simulink model "dynamic_simulation_synth_admittance_alone_2020a"  (R2020a)
settings: Solver=FixedStepAuto  StartTime=time_start  StopTime=time_end  FixedStep=dt  RelTol=1e-3
values from neighbouring files (symbols this model uses):
  B = 10    [hinfCostFunc.m]    (also in hinf_analysis_z.m; hinf_cmd_lmi.m = [zeros(4,2); Sigma.B]; init_rob_synth_sim.m; muCostFunc.m = 11)
  dth0 = dq0    [init_rob_synth_sim.m]
  dv = 1e-3    (= 0.001)    [init_rob_synth_sim.m]
  Fc = Fs    [init_rob_synth_sim.m]
  Fs = [0.9, 1.3, 0.5]    [init_rob_synth_sim.m]
  Fv = diag([0.5,0.37,0.7])    [init_rob_synth_sim.m]
  K = 150    [hinfCostFunc.m]    (also in hinf_analysis_z.m; init_rob_synth_sim.m; muCostFunc.m = ureal('K',160,'Percentage',50); mu_analysis_z.m = ureal('K',160,'Percentage',50))
  Kv = [2500;1500;2000]/256    [init_rob_synth_sim.m]
  Kvi = [3000;900;1000]/65536    [init_rob_synth_sim.m]
  M = 0.45    [hinfCostFunc.m]    (also in hinf_analysis_z.m; init_rob_synth_sim.m; muCostFunc.m = 0.42; mu_analysis_z.m = 0.42)
  nu = [0.8554, 0.5780, 0.9997]    [init_rob_synth_sim.m]
  R = [156;100;71]    [init_rob_synth_sim.m]
  tau_0 = [1.0000; 0.6119; 0.8268]    [init_rob_synth_sim.m]
  tau_m = 1/(10*2*pi)    (= 0.0159154943092)    [hinfCostFunc.m]    (also in hinf_analysis_z.m; init_rob_synth_sim.m; muCostFunc.m; mu_analysis_z.m)
  Tc = [0.0335;0.0335;0.051]    [init_rob_synth_sim.m]
  th0 = theta_DH(2:4) - (q0 - KUKA_offset(2:4))    [init_rob_synth_sim.m]
  thmax = theta_DH - (qmin - KUKA_offset)    [init_rob_synth_sim.m]
  thmin = theta_DH - (qmax - KUKA_offset)    [init_rob_synth_sim.m]
  W1 = 1/makeweight(1e-6,[2*pi*fc_w1,1],g_w1,0,2)    [hinfCostFunc.m]    (also in hinf_analysis_z.m = 1/makeweight(1e-6,[2*pi*fc_s,1],2,0,2); init_rob_synth_sim.m = makeweight(1.5,[2*pi*3,1],0); muCostFunc.m; mu_analysis_z.m = 1/makeweight(1e-6,[2*pi*x(1),1],x(3),0,2))
  W3 = makeweight(0,[2*pi*0.5,1],1.5)    [init_rob_synth_sim.m]    (also in mu_analysis_z.m = 1/makeweight(10^(33.4/20),[2*pi*fc_w3,10],0.1))
  W4 = makeweight(0,[2*pi*1,1],1.5)*makeweight(1.5,[2*pi*1,1],0)    [init_rob_synth_sim.m]
libraries: simulink x1
settings Model: Creator=fortineau_vin  LastModifiedBy=fortineau_vin
settings DataIOCC: ReturnWorkspaceOutputs=off
settings DebuggingCC: ArithmeticOperatorsInVariantConditions=warning
settings SFSimCC: SimUseLocalCustomCode=off  CustomCodeUndefinedFunction=UseInterfaceOnly
settings RTWCC: RTWUseLocalCustomCode=off

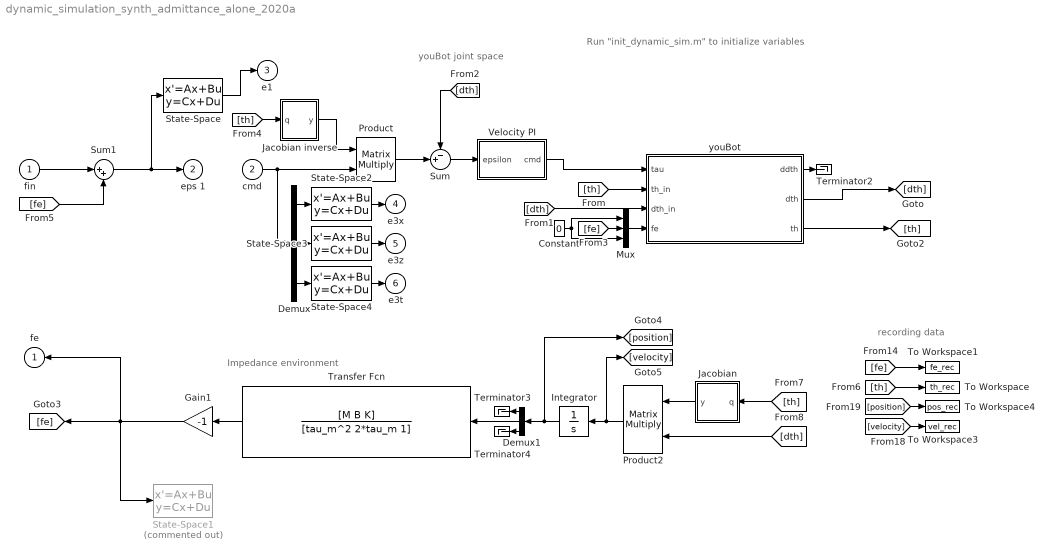
== system dynamic_simulation_synth_admittance_alone_2020a ==
  note: recording data
  note: Run "init_dynamic_sim.m" to initialize variables
  note: youBot joint space
  note: Impedance environment
  fin : Inport  PortDimensions=1
  cmd : Inport  Port=2  PortDimensions=3
  Constant : Constant  Value=0
  Demux : Demux  Outputs=3
  Demux1 : Demux  Outputs=3
  Gain1 : Gain  Gain=-1
  Integrator : Integrator
  Jacobian : MATLAB Function  TreatAsAtomicUnit=on
  Jacobian inverse : MATLAB Function  TreatAsAtomicUnit=on
  Mux : Mux  Inputs=3
  Product : Product  Multiplication=Matrix(*)
  Product2 : Product  Multiplication=Matrix(*)
  State-Space : StateSpace  A=W1.A  B=W1.B  C=W1.C  D=W1.D  InitialCondition=0
  State-Space1 : StateSpace  Commented=on  A=W4.A  B=W4.B  C=W4.C  D=W4.D  InitialCondition=0
  State-Space2 : StateSpace  A=W3.A  B=W3.B  C=W3.C  D=W3.D  InitialCondition=0
  State-Space3 : StateSpace  A=W3.A  B=W3.B  C=W3.C  D=W3.D  InitialCondition=0
  State-Space4 : StateSpace  A=W3.A  B=W3.B  C=W3.C  D=W3.D  InitialCondition=0
  Sum : Sum  Inputs=-+|
  Sum1 : Sum  Inputs=|++
  Terminator2 : Terminator
  Terminator3 : Terminator
  Terminator4 : Terminator
  To Workspace : ToWorkspace  VariableName=th_rec  SaveFormat=Structure  SampleTime=1e-3
      settings: Save2DSignal=2-D array (concatenate along first dimension)
  To Workspace1 : ToWorkspace  VariableName=fe_rec  SaveFormat=Structure  SampleTime=1e-3
      settings: Save2DSignal=2-D array (concatenate along first dimension)
  To Workspace3 : ToWorkspace  VariableName=vel_rec  SaveFormat=Structure  SampleTime=1e-3
      settings: Save2DSignal=2-D array (concatenate along first dimension)
  To Workspace4 : ToWorkspace  VariableName=pos_rec  SaveFormat=Structure  SampleTime=1e-3
      settings: Save2DSignal=2-D array (concatenate along first dimension)
  Transfer Fcn : TransferFcn  Numerator=[M B K]  Denominator=[tau_m^2 2*tau_m 1]
  Velocity PI : Subsystem
  youBot : Subsystem
  fe : Outport  PortDimensions=1
  eps 1 : Outport  Port=2
  e1 : Outport  Port=3  PortDimensions=1
  e3x : Outport  Port=4  PortDimensions=1
  e3z : Outport  Port=5  PortDimensions=1
  e3t : Outport  Port=6  PortDimensions=1
  wires:
  Sum/1 -> Velocity PI/1(epsilon)
  [dth] -> Sum/1
  Product/1 -> Sum/2
  [th] -> Jacobian inverse/1(q)
  [th] -> To Workspace/1
  [fe] -> To Workspace1/1
  [th] -> youBot/2(th_in)
  [dth] -> youBot/3(dth_in)
  youBot/1(ddth) -> Terminator2/1
  youBot/2(dth) -> [dth]
  youBot/3(th) -> [th]
  [velocity] -> To Workspace3/1
  [position] -> To Workspace4/1
  cmd/1 -> Demux/1, Product/2
  Jacobian inverse/1(y) -> Product/1
  Velocity PI/1(cmd) -> youBot/1(tau)
  [fe] -> Sum1/2
  [fe] -> Mux/2
  Sum1/1 -> State-Space/1, eps 1/1
  fin/1 -> Sum1/1
  [th] -> Jacobian/1(q)
  [dth] -> Product2/2
  Jacobian/1(y) -> Product2/1
  Transfer Fcn/1 -> Gain1/1
  Integrator/1 -> Demux1/1, [position]
  Product2/1 -> [velocity], Integrator/1
  State-Space/1 -> e1/1
  State-Space2/1 -> e3x/1
  Demux1/1 -> Terminator3/1
  Demux1/3 -> Terminator4/1
  Demux/1 -> State-Space2/1
  Demux/2 -> State-Space3/1
  Demux/3 -> State-Space4/1
  State-Space4/1 -> e3t/1
  State-Space3/1 -> e3z/1
  Demux1/2 -> Transfer Fcn/1
  Gain1/1 -> State-Space1/1, fe/1, [fe]
  Mux/1 -> youBot/4(fe)
  Constant/1 -> Mux/1, Mux/3

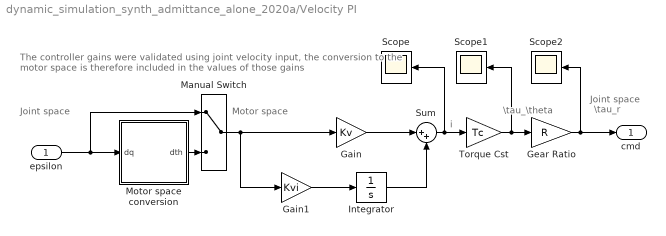
== system dynamic_simulation_synth_admittance_alone_2020a/Velocity PI ==
  note: The controller gains were validated using joint velocity input, the conversion to
      | the motor space is therefore included in the values of those gains
  note: \tau_\theta
  note: i
  note: Motor space
  note: Joint space
  note: \tau_r
  note: Joint space
  epsilon : Inport
  Gain : Gain  Gain=Kv
  Gain1 : Gain  Gain=Kvi
  Gear Ratio : Gain  Gain=R
  Integrator : Integrator
  Manual Switch : ManualSwitch
  Motor space conversion : Subsystem
  Scope : Scope
  Scope1 : Scope
  Scope2 : Scope
  Sum : Sum  Inputs=|++
  Torque Cst : Gain  Gain=Tc
  cmd : Outport  VectorParamsAs1DForOutWhenUnconnected=off
  wires:
  Gain/1 -> Sum/1
  Integrator/1 -> Sum/2
  Gear Ratio/1 -> Scope2/1, cmd/1
  Sum/1 -> Scope/1, Torque Cst/1
  Torque Cst/1 -> Scope1/1, Gear Ratio/1
  epsilon/1 -> Manual Switch/1, Motor space conversion/1(dq)
  Motor space conversion/1(dth) -> Manual Switch/2
  Manual Switch/1 -> Gain/1, Gain1/1
  Gain1/1 -> Integrator/1

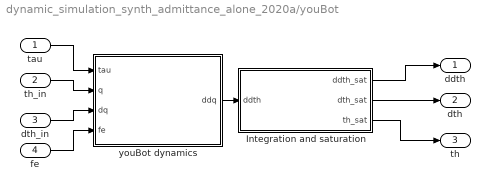
== system dynamic_simulation_synth_admittance_alone_2020a/youBot ==
  tau : Inport
  th_in : Inport  Port=2
  dth_in : Inport  Port=3
  fe : Inport  Port=4
  Integration and saturation : Subsystem
  youBot dynamics : Subsystem
  ddth : Outport  VectorParamsAs1DForOutWhenUnconnected=off
  dth : Outport  Port=2  VectorParamsAs1DForOutWhenUnconnected=off
  th : Outport  Port=3  VectorParamsAs1DForOutWhenUnconnected=off
  wires:
  tau/1 -> youBot dynamics/1(tau)
  youBot dynamics/1(ddq) -> Integration and saturation/1(ddth)
  dth_in/1 -> youBot dynamics/3("dq ")
  th_in/1 -> youBot dynamics/2("q ")
  fe/1 -> youBot dynamics/4(fe)
  Integration and saturation/3(th_sat) -> th/1
  Integration and saturation/1(ddth_sat) -> ddth/1
  Integration and saturation/2(dth_sat) -> dth/1

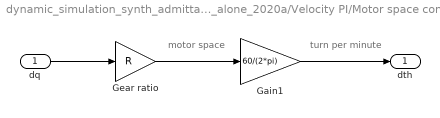
== system dynamic_simulation_synth_admittance_alone_2020a/Velocity PI/Motor space conversion ==
  note: motor space
  note: turn per minute
  dq : Inport
  Gain1 : Gain  Gain=60/(2*pi)
  Gear ratio : Gain  Gain=R
  dth : Outport  VectorParamsAs1DForOutWhenUnconnected=off
  wires:
  dq/1 -> Gear ratio/1
  Gear ratio/1 -> Gain1/1
  Gain1/1 -> dth/1

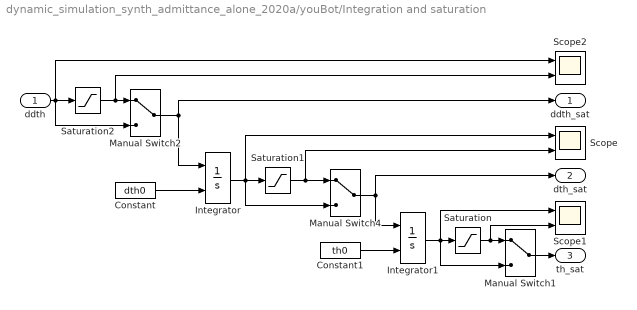
== system dynamic_simulation_synth_admittance_alone_2020a/youBot/Integration and saturation ==
  ddth : Inport
  Constant : Constant  Value=dth0
  Constant1 : Constant  Value=th0
  Integrator : Integrator  InitialConditionSource=external
  Integrator1 : Integrator  InitialConditionSource=external
  Manual Switch1 : ManualSwitch
  Manual Switch2 : ManualSwitch
  Manual Switch4 : ManualSwitch
  Saturation : Saturate  UpperLimit=thmax(2:4)'  LowerLimit=thmin(2:4)'
  Saturation1 : Saturate  UpperLimit=[2.685122; 4.188790; 5.899705]  LowerLimit=[-2.685122; -4.188790; -5.899705]
  Saturation2 : Saturate  UpperLimit=[10;10;10]  LowerLimit=[-10;-10;-10]
  Scope : Scope  NumInputPorts=2
  Scope1 : Scope  NumInputPorts=2
  Scope2 : Scope  NumInputPorts=2
  ddth_sat : Outport  VectorParamsAs1DForOutWhenUnconnected=off
  dth_sat : Outport  Port=2  VectorParamsAs1DForOutWhenUnconnected=off
  th_sat : Outport  Port=3  VectorParamsAs1DForOutWhenUnconnected=off
  wires:
  Manual Switch2/1 -> ddth_sat/1, Integrator/1
  Manual Switch1/1 -> th_sat/1
  Manual Switch4/1 -> Integrator1/1, dth_sat/1
  ddth/1 -> Scope2/1, Manual Switch2/2, Saturation2/1
  Saturation2/1 -> Scope2/2, Manual Switch2/1
  Saturation1/1 -> Scope/2, Manual Switch4/1
  Saturation/1 -> Scope1/2, Manual Switch1/1
  Constant/1 -> Integrator/2
  Integrator/1 -> Scope/1, Manual Switch4/2, Saturation1/1
  Integrator1/1 -> Scope1/1, Manual Switch1/2, Saturation/1
  Constant1/1 -> Integrator1/2

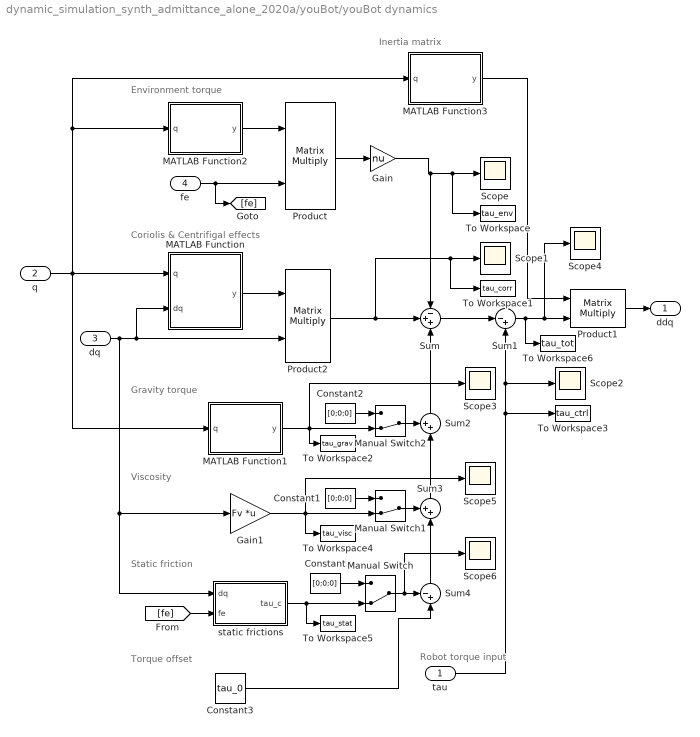
== system dynamic_simulation_synth_admittance_alone_2020a/youBot/youBot dynamics ==
  note: Coriolis & Centrifigal effects
  note: Gravity torque
  note: Environment torque
  note: Robot torque input
  note: Inertia matrix
  note: Viscosity
  note: Static friction
  note: Torque offset
  tau : Inport
  "q " : Inport  Port=2
  "dq " : Inport  Port=3
  fe : Inport  Port=4
  Constant : Constant  Value=[0;0;0]
  Constant1 : Constant  Value=[0;0;0]
  Constant2 : Constant  Value=[0;0;0]
  Constant3 : Constant  Value=tau_0
  Gain : Gain  Gain=nu
  Gain1 : Gain  Gain=Fv  Multiplication=Matrix(K*u)
  MATLAB Function : MATLAB Function  TreatAsAtomicUnit=on
  MATLAB Function1 : MATLAB Function  TreatAsAtomicUnit=on
  MATLAB Function2 : MATLAB Function  TreatAsAtomicUnit=on
  MATLAB Function3 : MATLAB Function  TreatAsAtomicUnit=on
  Manual Switch : ManualSwitch  CurrentSetting=0
  Manual Switch1 : ManualSwitch  CurrentSetting=0
  Manual Switch2 : ManualSwitch  CurrentSetting=0
  Product : Product  Multiplication=Matrix(*)
  Product1 : Product  Multiplication=Matrix(*)
  Product2 : Product  Multiplication=Matrix(*)
  Scope{,1..6} (7 alike) : Scope
  Sum : Sum  Inputs=-++
  Sum1 : Sum  Inputs=|-+
  Sum2 : Sum  Inputs=++|
  Sum3 : Sum  Inputs=++|
  Sum4 : Sum  Inputs=-+|
  To Workspace : ToWorkspace  VariableName=tau_env  SaveFormat=Timeseries  SampleTime=-1
  To Workspace1 : ToWorkspace  VariableName=tau_corr  SaveFormat=Timeseries  SampleTime=-1
  To Workspace2 : ToWorkspace  VariableName=tau_grav  SaveFormat=Timeseries  SampleTime=-1
  To Workspace3 : ToWorkspace  VariableName=tau_ctrl  SaveFormat=Timeseries  SampleTime=-1
  To Workspace4 : ToWorkspace  VariableName=tau_visc  SaveFormat=Timeseries  SampleTime=-1
  To Workspace5 : ToWorkspace  VariableName=tau_stat  SaveFormat=Timeseries  SampleTime=-1
  To Workspace6 : ToWorkspace  VariableName=tau_tot  SaveFormat=Timeseries  SampleTime=-1
  static frictions : Subsystem
  ddq : Outport  VectorParamsAs1DForOutWhenUnconnected=off
  wires:
  "dq "/1 -> Product2/2, MATLAB Function/2(dq), static frictions/1(dq), Gain1/1
  "q "/1 -> MATLAB Function/1(q), MATLAB Function2/1(q), MATLAB Function3/1(q), MATLAB Function1/1(q)
  Product/1 -> Gain/1
  Product1/1 -> ddq/1
  MATLAB Function1/1(y) -> Scope3/1, Manual Switch2/2, To Workspace2/1
  Sum/1 -> Sum1/1
  Product2/1 -> Scope1/1, To Workspace1/1, Sum/2
  MATLAB Function/1(y) -> Product2/1
  MATLAB Function2/1(y) -> Product/1
  fe/1 -> Product/2, [fe]
  MATLAB Function3/1(y) -> Product1/1
  Sum1/1 -> To Workspace6/1, Scope4/1, Product1/2
  tau/1 -> To Workspace3/1, Scope2/1, Sum1/2
  Gain/1 -> Scope/1, To Workspace/1, Sum/1
  Sum2/1 -> Sum/3
  Gain1/1 -> Manual Switch1/2, Scope5/1, To Workspace4/1
  [fe] -> static frictions/2(fe)
  Sum3/1 -> Sum2/2
  static frictions/1(tau_c) -> To Workspace5/1, Manual Switch/2
  Constant/1 -> Manual Switch/1
  Constant1/1 -> Manual Switch1/1
  Manual Switch1/1 -> Sum3/1
  Manual Switch2/1 -> Sum2/1
  Constant2/1 -> Manual Switch2/1
  Sum4/1 -> Sum3/2
  Manual Switch/1 -> Scope6/1, Sum4/1
  Constant3/1 -> Sum4/2

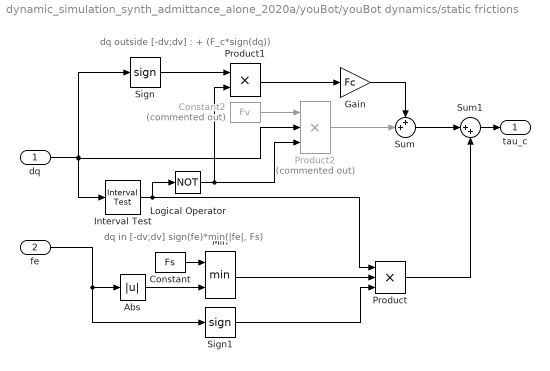
== system dynamic_simulation_synth_admittance_alone_2020a/youBot/youBot dynamics/static frictions ==
  note: dq in [-dv;dv]
      |
      | sign(fe)*min(|fe|, Fs)
  note: dq outside [-dv;dv] : + (F_c*sign(dq))
  dq : Inport
  fe : Inport  Port=2
  Abs : Abs
  Constant : Constant  Value=Fs
  Constant2 : Constant  Commented=on  Value=Fv
  Gain : Gain  Gain=Fc
  Interval Test : simulink/Logic and Bit Operations/Interval Test  IntervalClosedRight=on  uplimit=dv  IntervalClosedLeft=on  lowlimit=-dv  OutDataTypeStr=boolean
  Logical Operator : Logic  Operator=NOT  AllPortsSameDT=off  OutDataTypeStr=boolean
  Min : MinMax  Inputs=2
  Product : Product  Inputs=3
  Product1 : Product
  Product2 : Product  Commented=on  Inputs=3
  Sign : Signum
  Sign1 : Signum
  Sum : Sum  Inputs=++|
  Sum1 : Sum  Inputs=|++
  tau_c : Outport  VectorParamsAs1DForOutWhenUnconnected=off
  wires:
  Sum1/1 -> tau_c/1
  Interval Test/1 -> Logical Operator/1, Product/1
  fe/1 -> Sign1/1, Abs/1
  Abs/1 -> Min/2
  Constant/1 -> Min/1
  Min/1 -> Product/2
  Sign1/1 -> Product/3
  Logical Operator/1 -> Product1/2, Product2/3
  dq/1 -> Sign/1, Product2/2, Interval Test/1
  Constant2/1 -> Product2/1
  Product2/1 -> Sum/2
  Product1/1 -> Gain/1
  Sum/1 -> Sum1/1
  Product/1 -> Sum1/2
  Sign/1 -> Product1/1
  Gain/1 -> Sum/1

== matlab function dynamic_simulation_synth_admittance_alone_2020a/youBot/youBot dynamics/MATLAB Function ==
  data: q input; y output; dq input
function y = C_sim(q,dq)
q2 = q(2);
q3 = q(3);
dq1 = dq(1);
dq2 = dq(2);
dq3 = dq(3);
y = C_3DOF(dq1,dq2,dq3,q2,q3);

== matlab function dynamic_simulation_synth_admittance_alone_2020a/youBot/youBot dynamics/MATLAB Function2 ==
  data: q input; y output
function y = tJ_sim(q)
q1 = q(1);
q2 = q(2);
q3 = q(3);
y = J0E_3DOF(q1,q2,q3)';

== matlab function dynamic_simulation_synth_admittance_alone_2020a/youBot/youBot dynamics/MATLAB Function3 ==
  data: q input; y output
function y = iM_sim(q)
q2 = q(2);
q3 = q(3);
y = iM_3DOF(q2,q3);

== matlab function dynamic_simulation_synth_admittance_alone_2020a/Jacobian inverse ==
  data: q input; y output
function y = iJ(q)
q1 = q(1);
q2 = q(2);
q3 = q(3);
y = iJ0E_3DOF(q1,q2,q3);

== matlab function dynamic_simulation_synth_admittance_alone_2020a/Jacobian ==
  data: q input; y output
function y = J(q)
q1 = q(1);
q2 = q(2);
q3 = q(3);
y = J0E_3DOF(q1,q2,q3);

== matlab function dynamic_simulation_synth_admittance_alone_2020a/youBot/youBot dynamics/MATLAB Function1 ==
  data: q input; y output
function y = G_sim(q)
q1 = q(1);
q2 = q(2);
q3 = q(3);
y = G_3DOF(q1,q2,q3);
